simulink model "afe_abc_inv_psm"  (R2025b)
settings: Solver=ode1  StartTime=0.0  StopTime=simlength  FixedStep=tc  MaxStep=tc
values from neighbouring files (symbols this model uses):
  Adrso = eye(2) + Arso*ts_afe    [init_model.m]
  afe_pwm_phase_shift_mod1 = 0    [init_model.m]
  afe_pwm_phase_shift_mod2 = 0    [init_model.m]
  Aresd = eye(2) + Ares*ts_afe    [init_model.m]
  Bresd = Bres*ts_afe    [init_model.m]
  Cresd = Cres    [init_model.m]
  Crso = [1 0]    [init_model.m]
  CTRPIFF_CLIP_RELEASE = 0.001    [init_model.m]
  deepNEGeta = 0.5    [init_model.m]
  deepNEGxi = 0    [init_model.m]
  deepPOSxi = 0.5    [init_model.m]
  emf_fb_p = 0.2    [init_model.m]
  emf_fb_p_ccaller_1 = emf_fb_p    (= 0.2)    [init_model.m]
  emf_fb_p_ccaller_2 = emf_fb_p    (= 0.2)    [init_model.m]
  emf_p = emf_fb_p*4/10    (= 0.08)    [init_model.m]
  emf_p_ccaller_1 = emf_fb_p_ccaller_1*4/10    (= 0.08)    [init_model.m]
  emf_p_ccaller_2 = emf_fb_p_ccaller_2*4/10    (= 0.08)    [init_model.m]
  g0_161Hz = fcut_161Hz_flt * ts_afe * 2*pi    (= 0.126449104307)    [init_model.m]
  g0_1Hz = fcut_1Hz_flt * ts_afe * 2*pi    (= 0.000785398163397)    [init_model.m]
  g0_500Hz = fcut_500Hz_flt * ts_afe * 2*pi    (= 0.392699081699)    [init_model.m]
  g1_161Hz = 1 - g0_161Hz    (= 0.873550895693)    [init_model.m]
  g1_1Hz = 1 - g0_1Hz    (= 0.999214601837)    [init_model.m]
  g1_500Hz = 1 - g0_500Hz    (= 0.607300918301)    [init_model.m]
  i_grid_neg_eta_lim = 0.5    [init_model.m]
  i_grid_neg_eta_red_lim = 0.1    [init_model.m]
  i_grid_neg_xi_lim = 0.5    [init_model.m]
  i_grid_neg_xi_red_lim = 0.1    [init_model.m]
  i_grid_pos_eta_lim = 1    [init_model.m]
  i_grid_pos_eta_red_lim = 0.1    [init_model.m]
  id_lim = 0.35    [init_model.m]
  ieta_neg_ref_lim = 0.5    [init_model.m]
  ieta_pos_ref_lim = 1.0    (= 1)    [init_model.m]
  Igrid_phase_normalization_factor = 250e3/Vphase2/3/0.9*sqrt(2)    [init_model.m]
  inv_pwm_phase_shift_mod1 = 0    [init_model.m]
  iq_lim = 1.4    [init_model.m]
  ixi_pos_ref_lim = 1.6    [init_model.m]
  k_frt_ref = 2    [init_model.m]
  kg = Kobs(1)    [init_model.m]
  ki_afe = 45    [init_model.m]
  ki_align = 0.1    [init_model.m]
  ki_i = 18    [init_model.m]
  ki_rc_neg_grid = ki_rc_grid    (= 35)    [init_model.m]
  ki_rc_pos_grid = ki_rc_grid    (= 35)    [init_model.m]
  ki_vs = 35    [init_model.m]
  ki_w = 18    [init_model.m]
  kp_afe = 0.6    [init_model.m]
  kp_align = 0.6    [init_model.m]
  kp_i = 0.25    [init_model.m]
  kp_rc_neg_grid = kp_rc_grid    (= 0.35)    [init_model.m]
  kp_rc_pos_grid = kp_rc_grid    (= 0.35)    [init_model.m]
  kp_vs = 0.85    [init_model.m]
  kp_w = 2.5    [init_model.m]
  kw = Kobs(2)    [init_model.m]
  l1 = Kd(2)    [init_model.m]
  l2 = Kd(1)    [init_model.m]
  Ldrso = acker(Adrso',Crso',polesdrso)'    [init_model.m]
  lim_down_align = -0.2    [init_model.m]
  lim_up_align = 0.2    [init_model.m]
  mavarage_filter_frequency_base_order = 2    [init_model.m]
  motorc_m_scale = 2/3*Vdc_bez/ubez    [init_model.m]
  n1 = rms_perios/f_grid/ts_afe    [init_model.m]
  n10 = rms_perios/f_grid/ts_afe    [init_model.m]
  number_of_modules = 2    [init_model.m]
  omega_m_sim = omega_m_bez    [init_model.m]
  pll_i1 = 80    [init_model.m]
  pll_i1_ddsrt = pll_i1/2    (= 40)    [init_model.m]
  pll_p = 1    [init_model.m]
  pll_p_ddsrt = pll_p/2    (= 0.5)    [init_model.m]
  pll_p_frt = 0.2    [init_model.m]
  settle_time = 0.15    [init_model.m]
  simlength = 2    [init_model.m]
  start_time_LVRT = 2.0    (= 2)    [init_model.m]
  tc = ts_afe/200    (= 6.25e-07)    [init_model.m]
  time_aux_power_supply_fault = 1e3    (= 1000)    [init_model.m]
  time_gain_afe_module_1 = 1.0    (= 1)    [init_model.m]
  time_gain_afe_module_2 = 1.0    (= 1)    [init_model.m]
  time_gain_inv_module_1 = 1.0    (= 1)    [init_model.m]
  time_gain_inv_module_2 = 1.0    (= 1)    [init_model.m]
  time_phase_fault = 1e3    (= 1000)    [init_model.m]
  time_start_motor_control = 0.035    [init_model.m]
  transmission_delay = 125e-6*2    (= 0.00025)    [init_model.m]
  ts_afe = 1/fPWM_AFE/2    (= 0.000125)    [init_model.m]
  ts_inv = 1/fPWM_INV/2    (= 0.000125)    [init_model.m]
  Vdc_norm_ref = Vdc_ref/Vdc_nom    [init_model.m]
  Vdc_ref = 1070    [init_model.m]
  Vgrid_phase_normalization_factor = Vphase2*sqrt(2)    [init_model.m]
  w_grid = 2*pi*f_grid    [init_model.m]
undefined symbols (not defined in the file or in its folder): Amplitude_U, Amplitude_V, Amplitude_W, end_time_LVRT, ibez, La, Lb, Ld_norm, Lq_norm, Ls_norm, magnitude, omega_bez, omega_grid_emulator_nom, omega_grid_nom, omega_m_bez, Phase_shift, psi_bez, psi_m, psi_m_norm, rpm_base, rpm_bez, Rs, Rs_norm, t_ramp, tau_bez, torque_base, ubez, ugrid_factor, V_phase_normalization_factor, Vdc_bez, Vemu_ref_norm, vn_eta_pu, vn_xi_pu, vp_xi_pu
libraries: fl_lib x215, nesl_utility x107, simulink x22, cstblocks x20, threephase_inductor_lib x4, three_phase_pwm_modulator x4, single_phase_transformer_lib x3, power_meter_iec x1, flexshaft_lib x1, psm x1
(part 2 of 18)

== system afe_abc_inv_psm/afe_abc_inv_psm_mod1/brake ==
  Constant1 : Constant  Value=Vdc_ref
  Current Sensor3 : fl_lib/Electrical/Electrical Sensors/Current Sensor
  Integrator : Integrator
  MATLAB Function : MATLAB Function  TreatAsAtomicUnit=on  SystemSampleTime=ts_afe
  PS-Simulink Converter : nesl_utility/PS-Simulink Converter  PhysicalDomain=network_engine_domain  SubClassName=ps_output  LeftPortType=input  RightPortType=output  PseudoPeriodic=off  Frequencies=[]  VectorFormat=1-D array  Unit=V  AffineConversion=off
  Product : Product
  Product6 : Product
  Rbrake mod1 : Scope  NumInputPorts=2
      settings: SampleTime=tc  ActiveDisplayYMinimum=1.4840277431149421E-9  ActiveDisplayYMaximum=1.4991129263129132E-9  DataLoggingVariableName=ScopeData2
  Resistor : fl_lib/Electrical/Electrical Elements/Resistor  R=4 Ohm  i_specify=off  i_priority=None  i=0 A  i_nominal_specify=off  i_nominal_value=1  i_nominal_unit=A  v_specify=off  v_priority=None  v=0 V  v_nominal_specify=off  v_nominal_value=1  v_nominal_unit=V
  Simulink-PS Converter4 : nesl_utility/Simulink-PS Converter  PhysicalDomain=network_engine_domain  SubClassName=ps_input  LeftPortType=input  RightPortType=output  PseudoPeriodic=off  Frequencies=[]  NoiseDistribution=none  NoiseParameters=[]  Unit=1  AffineConversion=on  FilteringAndDerivatives=provide  SimscapeFilterOrder=1  InputFilterTimeConstant=0.001  UdotUserProvided=0
  Step : Step  Time=time_aux_power_supply_fault  Before=1  After=0  SampleTime=0
  To Workspace1 : ToWorkspace  VariableName=energy_Rbrake_sim_mod1  SampleTime=ts_afe
      settings: MaxDataPoints=Ns_afe
  To Workspace10 : ToWorkspace  VariableName=power_Rbrake_sim_mod1  SampleTime=ts_afe
      settings: MaxDataPoints=Ns_afe
  Unit Delay : UnitDelay  SampleTime=ts_afe  HasFrameUpgradeWarning=on
  Voltage Sensor : fl_lib/Electrical/Electrical Sensors/Voltage Sensor
  Voltage Sensor1 : fl_lib/Electrical/Electrical Sensors/Voltage Sensor
  ibrakeR : nesl_utility/PS-Simulink Converter  PhysicalDomain=network_engine_domain  SubClassName=ps_output  LeftPortType=input  RightPortType=output  PseudoPeriodic=off  Frequencies=[]  VectorFormat=1-D array  Unit=A  AffineConversion=off
  switch_5 : Subsystem
      settings: PortSchema="{\"entries\":[{\"content\":{\"sides\":[{\"content\":{\"connectorIds\":[\"LConn1\"]},\"type\":\"ConnectorPlacement.EquallySpacedRectSide\",\"uuid\":\"9277da8d-d460-43e6-8478-dd662f15d226\"},{\"content\":{\"connectorIds\":[],\"side\":\"RIGHT\"},\"type\":\"ConnectorPlacement.EquallySpacedRectSide\",\"uuid\":\"a7ece396-f1d9-4f4f-a05b-db1fc65d6e1d\"},{\"content\":{\"connectorIds\":[\"LConn2\"],\"side\":\"TOP\"},\"type\":\"ConnectorPlacement.EquallySpacedRectSide\",\"uuid\":\"fdd70777-e9cf-4317-afb6-cae87f75d5b0\"},{\"content\":{\"connectorIds\":[\"RConn1\"],\"side\":\"BOTTOM\"},\"type\":\"ConnectorPlacement.EquallySpacedRectSide\",\"uuid\":\"2353ed68-b1a1-4775-9ca9-31e268d5443b\"}]},\"type\":\"ConnectorPlacement.EquallySpacedConnector\",\"uuid\":\"d5479f4c-4e65-4791-adcb-73df11f88590\"}],\"packageUris\":[\"http://schema.mathworks.com/mf0/Connector/R2020b\"],\"version\":\"1.0\"}"
  switch_6 : Subsystem
      settings: PortSchema="{\"entries\":[{\"content\":{\"sides\":[{\"content\":{},\"type\":\"ConnectorPlacement.EquallySpacedRectSide\",\"uuid\":\"9277da8d-d460-43e6-8478-dd662f15d226\"},{\"content\":{\"side\":\"RIGHT\"},\"type\":\"ConnectorPlacement.EquallySpacedRectSide\",\"uuid\":\"a7ece396-f1d9-4f4f-a05b-db1fc65d6e1d\"},{\"content\":{\"connectorIds\":[\"LConn1\"],\"side\":\"TOP\"},\"type\":\"ConnectorPlacement.EquallySpacedRectSide\",\"uuid\":\"fdd70777-e9cf-4317-afb6-cae87f75d5b0\"},{\"content\":{\"connectorIds\":[\"RConn1\"],\"side\":\"BOTTOM\"},\"type\":\"ConnectorPlacement.EquallySpacedRectSide\",\"uuid\":\"2353ed68-b1a1-4775-9ca9-31e268d5443b\"}]},\"type\":\"ConnectorPlacement.EquallySpacedConnector\",\"uuid\":\"d5479f4c-4e65-4791-adcb-73df11f88590\"}],\"packageUris\":[\"http://schema.mathworks.com/mf0/Connector/R2020b\"],\"version\":\"1.0\"}"
  ubrakeR : nesl_utility/PS-Simulink Converter  PhysicalDomain=network_engine_domain  SubClassName=ps_output  LeftPortType=input  RightPortType=output  PseudoPeriodic=off  Frequencies=[]  VectorFormat=1-D array  Unit=V  AffineConversion=off
  dc(+) : PMIOPort  Side=Left
  dc(-) : PMIOPort  Port=2  Side=Left
  tag scope: energy_Rbrake_mod1=global, power_Rbrake_mod1=global
  wires:
  Constant1/1 -> MATLAB Function/2(udc_ref)
  PS-Simulink Converter/1 -> MATLAB Function/1(u)
  MATLAB Function/1(y) -> Unit Delay/1
  ibrakeR/1 -> Product/1  "ibrakeR"
  ubrakeR/1 -> Product/2  "ubrakeR"
  Product/1 -> [power_Rbrake_mod1], Integrator/1
  Integrator/1 -> [energy_Rbrake_mod1]
  [power_Rbrake_mod1] -> To Workspace10/1, Rbrake mod1/1  "power_Rbrake"
  [energy_Rbrake_mod1] -> To Workspace1/1, Rbrake mod1/2  "energy_Rbrake"
  Step/1 -> Product6/1
  Unit Delay/1 -> Product6/2
  Product6/1 -> Simulink-PS Converter4/1
  connections:
  dc(-)/RConn1 -- switch_5/RConn1 -- Voltage Sensor/RConn2
  Voltage Sensor1/LConn1 -- Resistor/LConn1 -- Current Sensor3/RConn2
  PS-Simulink Converter/LConn1 -- Voltage Sensor/RConn1
  switch_5/LConn1 -- Simulink-PS Converter4/RConn1
  switch_6/RConn1 -- Voltage Sensor1/RConn2 -- Resistor/RConn1 -- switch_5/LConn2
  Voltage Sensor/LConn1 -- Current Sensor3/LConn1 -- switch_6/LConn1 -- dc(+)/RConn1
  Current Sensor3/RConn1 -- ibrakeR/LConn1
  Voltage Sensor1/RConn1 -- ubrakeR/LConn1

== system afe_abc_inv_psm/afe_abc_inv_psm_mod1/inverter ==
  duvw : Inport
  Current Sensor : fl_lib/Electrical/Electrical Sensors/Current Sensor
  PS-Simulink Converter1 : nesl_utility/PS-Simulink Converter  PhysicalDomain=network_engine_domain  SubClassName=ps_output  LeftPortType=input  RightPortType=output  PseudoPeriodic=off  Frequencies=[]  VectorFormat=1-D array  Unit=A  AffineConversion=on
  PS-Simulink Converter4 : nesl_utility/PS-Simulink Converter  PhysicalDomain=network_engine_domain  SubClassName=ps_output  LeftPortType=input  RightPortType=output  PseudoPeriodic=off  Frequencies=[]  VectorFormat=1-D array  Unit=V  AffineConversion=on
  To Workspace : ToWorkspace  VariableName=idc_sim_mod1  SampleTime=tc
      settings: MaxDataPoints=Nc
  To Workspace1 : ToWorkspace  VariableName=udc_sim_mod1  SampleTime=tc
      settings: MaxDataPoints=Nc
  Transfer Fcn : TransferFcn  Denominator=[1e-2 1]
  Voltage Sensor : fl_lib/Electrical/Electrical Sensors/Voltage Sensor
  idc/udc : Scope  NumInputPorts=2
      settings: SampleTime=tc  ActiveDisplayYMinimum=-232.79227304961765  ActiveDisplayYMaximum=27.545875945686063
  inverter : Subsystem
  Udc(+) : PMIOPort  Side=Right
  Udc(-) : PMIOPort  Port=2  Side=Right
  us_u : PMIOPort  Port=3  Side=Left
  us_v : PMIOPort  Port=4  Side=Left
  us_w : PMIOPort  Port=5  Side=Left
  wires:
  PS-Simulink Converter4/1 -> To Workspace1/1, idc/udc/2  "udc"
  PS-Simulink Converter1/1 -> Transfer Fcn/1  "idc"
  Transfer Fcn/1 -> To Workspace/1, idc/udc/1  "idc_flt"
  duvw/1 -> inverter/1(duties_uvw)
  connections:
  PS-Simulink Converter4/LConn1 -- Voltage Sensor/RConn1
  us_u/RConn1 -- inverter/LConn1
  us_v/RConn1 -- inverter/LConn2
  us_w/RConn1 -- inverter/LConn3
  Voltage Sensor/RConn2 -- inverter/RConn2 -- Udc(-)/RConn1
  Current Sensor/LConn1 -- Udc(+)/RConn1
  Voltage Sensor/LConn1 -- inverter/RConn1 -- Current Sensor/RConn2
  PS-Simulink Converter1/LConn1 -- Current Sensor/RConn1

== system afe_abc_inv_psm/afe_abc_inv_psm_mod2/AFE_control ==
  afe_control : Subsystem
  dabc_out : Outport
  tag scope: local_time_corr_afe2=global
  wires:
  [ig_abc_pu_mod2] -> afe_control/3(ig_abc_pu)
  afe_control/1(duvw) -> dabc_out/1
  [vdc_pu_afe_mod2] -> afe_control/2(udc_pu)
  [is_abc_pu_mod2] -> afe_control/4(is_abc_pu)
  [ug_abc_pu_mod2] -> afe_control/1(ug_abc_pu)
  [TRGO_afe_module_2] -> afe_control/Trigger
  [time_afe_module_2] -> afe_control/5(local_time)
  [time_master] -> afe_control/6(master_time)
  afe_control/2(AFE2_local_time_corr) -> [local_time_corr_afe2]

== system afe_abc_inv_psm/afe_abc_inv_psm_mod2/INV_control ==
  inverter_control : Subsystem
  transmission_delay : UnitDelay  SampleTime=transmission_delay  HasFrameUpgradeWarning=on
  duvw_out : Outport
  tag scope: local_time_corr_inv2=global
  wires:
  inverter_control/1(duvw) -> duvw_out/1
  [vdc_pu_inv_mod2] -> inverter_control/2(udc_pu)
  [TRGO_inv_module_2] -> inverter_control/Trigger
  [is_uvw_pu_mod2] -> inverter_control/1(is_uvw)
  [time_inv_module_2] -> inverter_control/3(local_time)
  [time_master] -> inverter_control/4(master_time)
  inverter_control/2(INV2_local_time_corr) -> [local_time_corr_inv2]
  [master_torque_ref] -> transmission_delay/1
  transmission_delay/1 -> inverter_control/5(master_torque_ref)
  [theta_elec_psm] -> inverter_control/6(theta_elec_psm)

== system afe_abc_inv_psm/afe_abc_inv_psm_mod2/LCL_filter ==
  CFu1 : fl_lib/Electrical/Electrical Elements/Capacitor  c=CFu F  r=RCFu Ohm  g=0 1/Ohm  i_specify=off  i_priority=None  i=0 A  i_nominal_specify=off  i_nominal_value=1  i_nominal_unit=A  v_specify=off  v_priority=None  v=0 V  v_nominal_specify=off  v_nominal_value=1  v_nominal_unit=V  vc_specify=off  vc_priority=High  vc=0 V  vc_nominal_specify=off  vc_nominal_value=1  vc_nominal_unit=V
  CFu2 : fl_lib/Electrical/Electrical Elements/Capacitor  c=CFu F  r=RCFu Ohm  g=0 1/Ohm  i_specify=off  i_priority=None  i=0 A  i_nominal_specify=off  i_nominal_value=1  i_nominal_unit=A  v_specify=off  v_priority=None  v=0 V  v_nominal_specify=off  v_nominal_value=1  v_nominal_unit=V  vc_specify=off  vc_priority=High  vc=0 V  vc_nominal_specify=off  vc_nominal_value=1  vc_nominal_unit=V
  CFu3 : fl_lib/Electrical/Electrical Elements/Capacitor  c=CFu F  r=RCFu Ohm  g=0 1/Ohm  i_specify=off  i_priority=None  i=0 A  i_nominal_specify=off  i_nominal_value=1  i_nominal_unit=A  v_specify=off  v_priority=None  v=0 V  v_nominal_specify=off  v_nominal_value=1  v_nominal_unit=V  vc_specify=off  vc_priority=High  vc=0 V  vc_nominal_specify=off  vc_nominal_value=1  vc_nominal_unit=V
  Inductor : fl_lib/Electrical/Electrical Elements/Inductor  l=1e-6 H  r=0 Ohm  g=1e-9 1/Ohm  i_specify=on  i_priority=High  i=0 A  i_nominal_specify=off  i_nominal_value=1  i_nominal_unit=A  v_specify=off  v_priority=None  v=0 V  v_nominal_specify=off  v_nominal_value=1  v_nominal_unit=V  i_L_specify=off  i_L_priority=High  i_L=0 A  i_L_nominal_specify=off  i_L_nominal_value=1  i_L_nominal_unit=A
  Inductor1 : fl_lib/Electrical/Electrical Elements/Inductor  l=1e-6 H  r=0 Ohm  g=1e-9 1/Ohm  i_specify=on  i_priority=High  i=0 A  i_nominal_specify=off  i_nominal_value=1  i_nominal_unit=A  v_specify=off  v_priority=None  v=0 V  v_nominal_specify=off  v_nominal_value=1  v_nominal_unit=V  i_L_specify=off  i_L_priority=High  i_L=0 A  i_L_nominal_specify=off  i_L_nominal_value=1  i_L_nominal_unit=A
  Inductor2 : fl_lib/Electrical/Electrical Elements/Inductor  l=1e-6 H  r=0 Ohm  g=1e-9 1/Ohm  i_specify=on  i_priority=High  i=0 A  i_nominal_specify=off  i_nominal_value=1  i_nominal_unit=A  v_specify=off  v_priority=None  v=0 V  v_nominal_specify=off  v_nominal_value=1  v_nominal_unit=V  i_L_specify=off  i_L_priority=High  i_L=0 A  i_L_nominal_specify=off  i_L_nominal_value=1  i_L_nominal_unit=A
  threephase inductor : threephase_inductor_lib/threephase inductor  Lp=LFu1_AFE H  L0=LFu1_AFE_0 H  Rp=2.4e-3 Ohm  R0=0.8e-3 Ohm  Lls=5e-6 H  uu_1_specify=off  uu_1_priority=None  uu_1=0 V  uu_1_nominal_specify=off  uu_1_nominal_unit=V  uu_1_nominal_value=1  uv_1_specify=off  uv_1_priority=None  uv_1=0 V  uv_1_nominal_specify=off  uv_1_nominal_unit=V  uv_1_nominal_value=1  uw_1_specify=off  uw_1_priority=None  uw_1=0 V  uw_1_nominal_specify=off  uw_1_nominal_unit=V  uw_1_nominal_value=1  uu_2_specify=off  uu_2_priority=None  uu_2=0 V  uu_2_nominal_specify=off  uu_2_nominal_unit=V  uu_2_nominal_value=1  uv_2_specify=off  uv_2_priority=None  uv_2=0 V  uv_2_nominal_specify=off  uv_2_nominal_unit=V  uv_2_nominal_value=1  uw_2_specify=off  uw_2_priority=None  uw_2=0 V  uw_2_nominal_specify=off  uw_2_nominal_unit=V  uw_2_nominal_value=1  iu_specify=off  iu_priority=High  iu=0 A  iu_nominal_specify=off  iu_nominal_unit=A  iu_nominal_value=1  iv_specify=off  iv_priority=High  iv=0 A  iv_nominal_specify=off  iv_nominal_unit=A  iv_nominal_value=1  iw_specify=off  iw_priority=High  iw=0 A  iw_nominal_specify=off  iw_nominal_unit=A  iw_nominal_value=1
      settings: InternalSimscapePortConfiguration="{\"Bottom\":[],\"Left\":[{\"id\":\"up1\",\"label\":\"u1\",\"type\":\"foundation.electrical.electrical\"},{\"id\":\"vp1\",\"label\":\"v1\",\"type\":\"foundation.electrical.electrical\"},{\"id\":\"wp1\",\"label\":\"w1\",\"type\":\"foundation.electrical.electrical\"}],\"Right\":[{\"id\":\"up2\",\"label\":\"u2\",\"type\":\"foundation.electrical.electrical\"},{\"id\":\"vp2\",\"label\":\"v2\",\"type\":\"foundation.electrical.electrical\"},{\"id\":\"wp2\",\"label\":\"w2\",\"type\":\"foundation.electrical.electrical\"}],\"Top\":[]}"
  threephase_vi_measures_stack : Subsystem
  threephase_vi_measures_stack1 : Subsystem
  us_a : PMIOPort  Side=Left
  ug_a : PMIOPort  Port=2  Side=Right
  us_b : PMIOPort  Port=3  Side=Left
  ug_b : PMIOPort  Port=4  Side=Right
  us_c : PMIOPort  Port=5  Side=Left
  ug_c : PMIOPort  Port=6  Side=Right
  connections:
  ug_c/RConn1 -- threephase_vi_measures_stack1/RConn3
  ug_b/RConn1 -- threephase_vi_measures_stack1/RConn2
  ug_a/RConn1 -- threephase_vi_measures_stack1/RConn1
  Inductor2/LConn1 -- threephase inductor/RConn3
  Inductor1/LConn1 -- threephase inductor/RConn2
  threephase inductor/RConn1 -- Inductor/LConn1
  threephase_vi_measures_stack/RConn3 -- threephase inductor/LConn3
  threephase_vi_measures_stack/RConn2 -- threephase inductor/LConn2
  threephase_vi_measures_stack/RConn1 -- threephase inductor/LConn1
  threephase_vi_measures_stack/LConn3 -- us_c/RConn1
  threephase_vi_measures_stack/LConn2 -- us_b/RConn1
  threephase_vi_measures_stack/LConn1 -- us_a/RConn1
  CFu2/LConn1 -- threephase_vi_measures_stack1/LConn2 -- Inductor1/RConn1
  CFu3/LConn1 -- threephase_vi_measures_stack1/LConn3 -- Inductor2/RConn1
  CFu1/LConn1 -- threephase_vi_measures_stack1/LConn1 -- Inductor/RConn1
  CFu1/RConn1 -- CFu2/RConn1 -- CFu3/RConn1

== system afe_abc_inv_psm/afe_abc_inv_psm_mod2/L_filter ==
  Inductor : fl_lib/Electrical/Electrical Elements/Inductor  l=1e-6 H  r=0 Ohm  g=1e-9 1/Ohm  i_specify=off  i_priority=None  i=0 A  i_nominal_specify=off  i_nominal_value=1  i_nominal_unit=A  v_specify=off  v_priority=None  v=0 V  v_nominal_specify=off  v_nominal_value=1  v_nominal_unit=V  i_L_specify=off  i_L_priority=High  i_L=0 A  i_L_nominal_specify=off  i_L_nominal_value=1  i_L_nominal_unit=A
  Inductor1 : fl_lib/Electrical/Electrical Elements/Inductor  l=1e-6 H  r=0 Ohm  g=1e-9 1/Ohm  i_specify=off  i_priority=None  i=0 A  i_nominal_specify=off  i_nominal_value=1  i_nominal_unit=A  v_specify=off  v_priority=None  v=0 V  v_nominal_specify=off  v_nominal_value=1  v_nominal_unit=V  i_L_specify=off  i_L_priority=High  i_L=0 A  i_L_nominal_specify=off  i_L_nominal_value=1  i_L_nominal_unit=A
  Inductor2 : fl_lib/Electrical/Electrical Elements/Inductor  l=1e-6 H  r=0 Ohm  g=1e-9 1/Ohm  i_specify=off  i_priority=None  i=0 A  i_nominal_specify=off  i_nominal_value=1  i_nominal_unit=A  v_specify=off  v_priority=None  v=0 V  v_nominal_specify=off  v_nominal_value=1  v_nominal_unit=V  i_L_specify=off  i_L_priority=High  i_L=0 A  i_L_nominal_specify=off  i_L_nominal_value=1  i_L_nominal_unit=A
  threephase inductor : threephase_inductor_lib/threephase inductor  Lp=LFi H  L0=LFi_0 H  Rp=2.4e-3 Ohm  R0=0.8e-3 Ohm  Lls=5e-6 H  uu_1_specify=off  uu_1_priority=None  uu_1=0 V  uu_1_nominal_specify=off  uu_1_nominal_unit=V  uu_1_nominal_value=1  uv_1_specify=off  uv_1_priority=None  uv_1=0 V  uv_1_nominal_specify=off  uv_1_nominal_unit=V  uv_1_nominal_value=1  uw_1_specify=off  uw_1_priority=None  uw_1=0 V  uw_1_nominal_specify=off  uw_1_nominal_unit=V  uw_1_nominal_value=1  uu_2_specify=off  uu_2_priority=None  uu_2=0 V  uu_2_nominal_specify=off  uu_2_nominal_unit=V  uu_2_nominal_value=1  uv_2_specify=off  uv_2_priority=None  uv_2=0 V  uv_2_nominal_specify=off  uv_2_nominal_unit=V  uv_2_nominal_value=1  uw_2_specify=off  uw_2_priority=None  uw_2=0 V  uw_2_nominal_specify=off  uw_2_nominal_unit=V  uw_2_nominal_value=1  iu_specify=off  iu_priority=None  iu=0 A  iu_nominal_specify=off  iu_nominal_unit=A  iu_nominal_value=1  iv_specify=off  iv_priority=None  iv=0 A  iv_nominal_specify=off  iv_nominal_unit=A  iv_nominal_value=1  iw_specify=off  iw_priority=None  iw=0 A  iw_nominal_specify=off  iw_nominal_unit=A  iw_nominal_value=1
      settings: InternalSimscapePortConfiguration="{\"Bottom\":[],\"Left\":[{\"id\":\"up1\",\"label\":\"u1\",\"type\":\"foundation.electrical.electrical\"},{\"id\":\"vp1\",\"label\":\"v1\",\"type\":\"foundation.electrical.electrical\"},{\"id\":\"wp1\",\"label\":\"w1\",\"type\":\"foundation.electrical.electrical\"}],\"Right\":[{\"id\":\"up2\",\"label\":\"u2\",\"type\":\"foundation.electrical.electrical\"},{\"id\":\"vp2\",\"label\":\"v2\",\"type\":\"foundation.electrical.electrical\"},{\"id\":\"wp2\",\"label\":\"w2\",\"type\":\"foundation.electrical.electrical\"}],\"Top\":[]}"
  threephase_vi_measures_stack : Subsystem
  us_u : PMIOPort  Side=Left
  uu : PMIOPort  Port=2  Side=Right
  us_v : PMIOPort  Port=3  Side=Left
  uv : PMIOPort  Port=4  Side=Right
  us_w : PMIOPort  Port=5  Side=Left
  uw : PMIOPort  Port=6  Side=Right
  connections:
  Inductor2/RConn1 -- uw/RConn1
  Inductor1/RConn1 -- uv/RConn1
  Inductor/RConn1 -- uu/RConn1
  threephase inductor/RConn3 -- Inductor2/LConn1
  threephase inductor/RConn2 -- Inductor1/LConn1
  threephase inductor/RConn1 -- Inductor/LConn1
  threephase inductor/LConn3 -- threephase_vi_measures_stack/RConn3
  threephase inductor/LConn2 -- threephase_vi_measures_stack/RConn2
  threephase inductor/LConn1 -- threephase_vi_measures_stack/RConn1
  threephase_vi_measures_stack/LConn3 -- us_w/RConn1
  threephase_vi_measures_stack/LConn2 -- us_v/RConn1
  threephase_vi_measures_stack/LConn1 -- us_u/RConn1

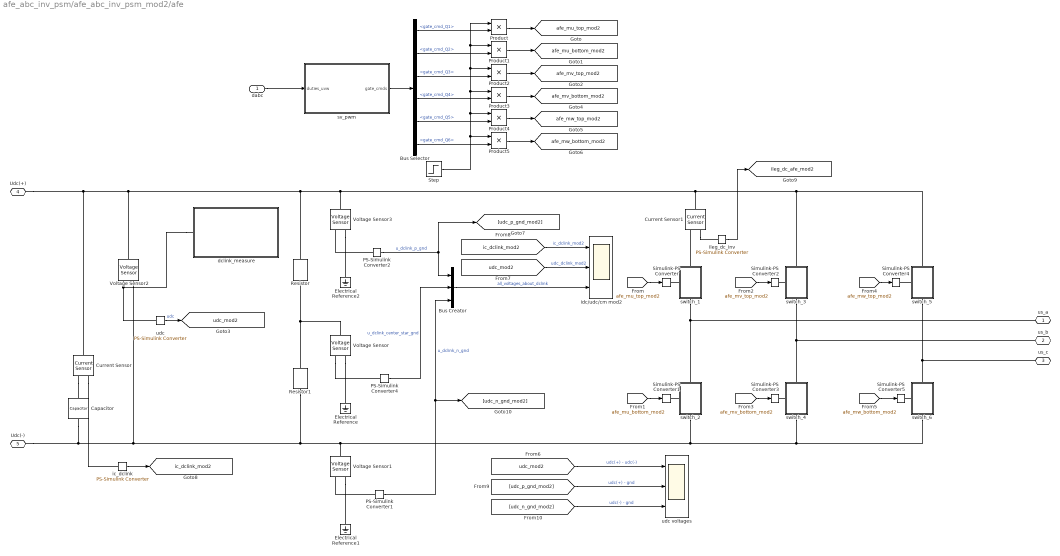
== system afe_abc_inv_psm/afe_abc_inv_psm_mod2/afe ==
  dabc : Inport
  Bus Creator : BusCreator  Inputs=3
  Bus Selector : BusSelector  OutputSignals=gate_cmd_Q1,gate_cmd_Q2,gate_cmd_Q3,gate_cmd_Q4,gate_cmd_Q5,gate_cmd_Q6
  Capacitor : fl_lib/Electrical/Electrical Elements/Capacitor  c=CFi F  r=0.2e-3 Ohm  g=0 1/Ohm  i_specify=off  i_priority=None  i=0 A  i_nominal_specify=off  i_nominal_value=1  i_nominal_unit=A  v_specify=on  v_priority=High  v=Vdc_bez V  v_nominal_specify=off  v_nominal_value=1  v_nominal_unit=V  vc_specify=on  vc_priority=High  vc=Vdc_bez V  vc_nominal_specify=off  vc_nominal_value=1  vc_nominal_unit=V
  Current Sensor : fl_lib/Electrical/Electrical Sensors/Current Sensor
  Current Sensor1 : fl_lib/Electrical/Electrical Sensors/Current Sensor
  Electrical Reference : fl_lib/Electrical/Electrical Elements/Electrical Reference
  Electrical Reference1 : fl_lib/Electrical/Electrical Elements/Electrical Reference
  Electrical Reference2 : fl_lib/Electrical/Electrical Elements/Electrical Reference
  PS-Simulink Converter1 : nesl_utility/PS-Simulink Converter  PhysicalDomain=network_engine_domain  SubClassName=ps_output  LeftPortType=input  RightPortType=output  PseudoPeriodic=off  Frequencies=[]  VectorFormat=1-D array  Unit=V  AffineConversion=on
  PS-Simulink Converter2 : nesl_utility/PS-Simulink Converter  PhysicalDomain=network_engine_domain  SubClassName=ps_output  LeftPortType=input  RightPortType=output  PseudoPeriodic=off  Frequencies=[]  VectorFormat=1-D array  Unit=V  AffineConversion=on
  PS-Simulink Converter4 : nesl_utility/PS-Simulink Converter  PhysicalDomain=network_engine_domain  SubClassName=ps_output  LeftPortType=input  RightPortType=output  PseudoPeriodic=off  Frequencies=[]  VectorFormat=1-D array  Unit=V  AffineConversion=on
  Product{,1..5} (6 alike) : Product
  Resistor : fl_lib/Electrical/Electrical Elements/Resistor  R=1e6 Ohm  i_specify=off  i_priority=None  i=0 A  i_nominal_specify=off  i_nominal_value=1  i_nominal_unit=A  v_specify=off  v_priority=None  v=0 V  v_nominal_specify=off  v_nominal_value=1  v_nominal_unit=V
  Resistor1 : fl_lib/Electrical/Electrical Elements/Resistor  R=1e6 Ohm  i_specify=off  i_priority=None  i=0 A  i_nominal_specify=off  i_nominal_value=1  i_nominal_unit=A  v_specify=off  v_priority=None  v=0 V  v_nominal_specify=off  v_nominal_value=1  v_nominal_unit=V
  Simulink-PS Converter{,1..5} (6 alike) : nesl_utility/Simulink-PS Converter  PhysicalDomain=network_engine_domain  SubClassName=ps_input  LeftPortType=input  RightPortType=output  PseudoPeriodic=off  Frequencies=[]  NoiseDistribution=none  NoiseParameters=[]  Unit=1  AffineConversion=off  FilteringAndDerivatives=provide  SimscapeFilterOrder=1  InputFilterTimeConstant=0.001  UdotUserProvided=0
  Step : Step  Time=time_aux_power_supply_fault  Before=1  After=0  SampleTime=0
  Voltage Sensor{,1..3} (4 alike) : fl_lib/Electrical/Electrical Sensors/Voltage Sensor
  dclink_measure : Subsystem
  ic_dclink : nesl_utility/PS-Simulink Converter  PhysicalDomain=network_engine_domain  SubClassName=ps_output  LeftPortType=input  RightPortType=output  PseudoPeriodic=off  Frequencies=[]  VectorFormat=1-D array  Unit=A  AffineConversion=on
  idc/udc/cm mod2 : Scope  NumInputPorts=3
      settings: SampleTime=tc  ActiveDisplayYMinimum=-429.54161859669227  ActiveDisplayYMaximum=384.63505854745779
  ileg_dc_inv : nesl_utility/PS-Simulink Converter  PhysicalDomain=network_engine_domain  SubClassName=ps_output  LeftPortType=input  RightPortType=output  PseudoPeriodic=off  Frequencies=[]  VectorFormat=1-D array  Unit=A  AffineConversion=on
  sv_pwm : Subsystem
  switch_1 : Subsystem
      settings: PortSchema="{\"entries\":[{\"content\":{\"sides\":[{\"content\":{\"connectorIds\":[\"LConn1\"]},\"type\":\"ConnectorPlacement.EquallySpacedRectSide\",\"uuid\":\"9277da8d-d460-43e6-8478-dd662f15d226\"},{\"content\":{\"connectorIds\":[],\"side\":\"RIGHT\"},\"type\":\"ConnectorPlacement.EquallySpacedRectSide\",\"uuid\":\"a7ece396-f1d9-4f4f-a05b-db1fc65d6e1d\"},{\"content\":{\"connectorIds\":[\"LConn2\"],\"side\":\"TOP\"},\"type\":\"ConnectorPlacement.EquallySpacedRectSide\",\"uuid\":\"fdd70777-e9cf-4317-afb6-cae87f75d5b0\"},{\"content\":{\"connectorIds\":[\"RConn1\"],\"side\":\"BOTTOM\"},\"type\":\"ConnectorPlacement.EquallySpacedRectSide\",\"uuid\":\"2353ed68-b1a1-4775-9ca9-31e268d5443b\"}]},\"type\":\"ConnectorPlacement.EquallySpacedConnector\",\"uuid\":\"d5479f4c-4e65-4791-adcb-73df11f88590\"}],\"packageUris\":[\"http://schema.mathworks.com/mf0/Connector/R2020b\"],\"version\":\"1.0\"}"
  switch_2 : Subsystem
      settings: PortSchema="{\"entries\":[{\"content\":{\"sides\":[{\"content\":{\"connectorIds\":[\"LConn1\"]},\"type\":\"ConnectorPlacement.EquallySpacedRectSide\",\"uuid\":\"9277da8d-d460-43e6-8478-dd662f15d226\"},{\"content\":{\"connectorIds\":[],\"side\":\"RIGHT\"},\"type\":\"ConnectorPlacement.EquallySpacedRectSide\",\"uuid\":\"a7ece396-f1d9-4f4f-a05b-db1fc65d6e1d\"},{\"content\":{\"connectorIds\":[\"LConn2\"],\"side\":\"TOP\"},\"type\":\"ConnectorPlacement.EquallySpacedRectSide\",\"uuid\":\"fdd70777-e9cf-4317-afb6-cae87f75d5b0\"},{\"content\":{\"connectorIds\":[\"RConn1\"],\"side\":\"BOTTOM\"},\"type\":\"ConnectorPlacement.EquallySpacedRectSide\",\"uuid\":\"2353ed68-b1a1-4775-9ca9-31e268d5443b\"}]},\"type\":\"ConnectorPlacement.EquallySpacedConnector\",\"uuid\":\"d5479f4c-4e65-4791-adcb-73df11f88590\"}],\"packageUris\":[\"http://schema.mathworks.com/mf0/Connector/R2020b\"],\"version\":\"1.0\"}"
  switch_3 : Subsystem
      settings: PortSchema="{\"entries\":[{\"content\":{\"sides\":[{\"content\":{\"connectorIds\":[\"LConn1\"]},\"type\":\"ConnectorPlacement.EquallySpacedRectSide\",\"uuid\":\"9277da8d-d460-43e6-8478-dd662f15d226\"},{\"content\":{\"connectorIds\":[],\"side\":\"RIGHT\"},\"type\":\"ConnectorPlacement.EquallySpacedRectSide\",\"uuid\":\"a7ece396-f1d9-4f4f-a05b-db1fc65d6e1d\"},{\"content\":{\"connectorIds\":[\"LConn2\"],\"side\":\"TOP\"},\"type\":\"ConnectorPlacement.EquallySpacedRectSide\",\"uuid\":\"fdd70777-e9cf-4317-afb6-cae87f75d5b0\"},{\"content\":{\"connectorIds\":[\"RConn1\"],\"side\":\"BOTTOM\"},\"type\":\"ConnectorPlacement.EquallySpacedRectSide\",\"uuid\":\"2353ed68-b1a1-4775-9ca9-31e268d5443b\"}]},\"type\":\"ConnectorPlacement.EquallySpacedConnector\",\"uuid\":\"d5479f4c-4e65-4791-adcb-73df11f88590\"}],\"packageUris\":[\"http://schema.mathworks.com/mf0/Connector/R2020b\"],\"version\":\"1.0\"}"
  switch_4 : Subsystem
      settings: PortSchema="{\"entries\":[{\"content\":{\"sides\":[{\"content\":{\"connectorIds\":[\"LConn1\"]},\"type\":\"ConnectorPlacement.EquallySpacedRectSide\",\"uuid\":\"9277da8d-d460-43e6-8478-dd662f15d226\"},{\"content\":{\"connectorIds\":[],\"side\":\"RIGHT\"},\"type\":\"ConnectorPlacement.EquallySpacedRectSide\",\"uuid\":\"a7ece396-f1d9-4f4f-a05b-db1fc65d6e1d\"},{\"content\":{\"connectorIds\":[\"LConn2\"],\"side\":\"TOP\"},\"type\":\"ConnectorPlacement.EquallySpacedRectSide\",\"uuid\":\"fdd70777-e9cf-4317-afb6-cae87f75d5b0\"},{\"content\":{\"connectorIds\":[\"RConn1\"],\"side\":\"BOTTOM\"},\"type\":\"ConnectorPlacement.EquallySpacedRectSide\",\"uuid\":\"2353ed68-b1a1-4775-9ca9-31e268d5443b\"}]},\"type\":\"ConnectorPlacement.EquallySpacedConnector\",\"uuid\":\"d5479f4c-4e65-4791-adcb-73df11f88590\"}],\"packageUris\":[\"http://schema.mathworks.com/mf0/Connector/R2020b\"],\"version\":\"1.0\"}"
  switch_5 : Subsystem
      settings: PortSchema="{\"entries\":[{\"content\":{\"sides\":[{\"content\":{\"connectorIds\":[\"LConn1\"]},\"type\":\"ConnectorPlacement.EquallySpacedRectSide\",\"uuid\":\"9277da8d-d460-43e6-8478-dd662f15d226\"},{\"content\":{\"connectorIds\":[],\"side\":\"RIGHT\"},\"type\":\"ConnectorPlacement.EquallySpacedRectSide\",\"uuid\":\"a7ece396-f1d9-4f4f-a05b-db1fc65d6e1d\"},{\"content\":{\"connectorIds\":[\"LConn2\"],\"side\":\"TOP\"},\"type\":\"ConnectorPlacement.EquallySpacedRectSide\",\"uuid\":\"fdd70777-e9cf-4317-afb6-cae87f75d5b0\"},{\"content\":{\"connectorIds\":[\"RConn1\"],\"side\":\"BOTTOM\"},\"type\":\"ConnectorPlacement.EquallySpacedRectSide\",\"uuid\":\"2353ed68-b1a1-4775-9ca9-31e268d5443b\"}]},\"type\":\"ConnectorPlacement.EquallySpacedConnector\",\"uuid\":\"d5479f4c-4e65-4791-adcb-73df11f88590\"}],\"packageUris\":[\"http://schema.mathworks.com/mf0/Connector/R2020b\"],\"version\":\"1.0\"}"
  switch_6 : Subsystem
      settings: PortSchema="{\"entries\":[{\"content\":{\"sides\":[{\"content\":{\"connectorIds\":[\"LConn1\"]},\"type\":\"ConnectorPlacement.EquallySpacedRectSide\",\"uuid\":\"9277da8d-d460-43e6-8478-dd662f15d226\"},{\"content\":{\"connectorIds\":[],\"side\":\"RIGHT\"},\"type\":\"ConnectorPlacement.EquallySpacedRectSide\",\"uuid\":\"a7ece396-f1d9-4f4f-a05b-db1fc65d6e1d\"},{\"content\":{\"connectorIds\":[\"LConn2\"],\"side\":\"TOP\"},\"type\":\"ConnectorPlacement.EquallySpacedRectSide\",\"uuid\":\"fdd70777-e9cf-4317-afb6-cae87f75d5b0\"},{\"content\":{\"connectorIds\":[\"RConn1\"],\"side\":\"BOTTOM\"},\"type\":\"ConnectorPlacement.EquallySpacedRectSide\",\"uuid\":\"2353ed68-b1a1-4775-9ca9-31e268d5443b\"}]},\"type\":\"ConnectorPlacement.EquallySpacedConnector\",\"uuid\":\"d5479f4c-4e65-4791-adcb-73df11f88590\"}],\"packageUris\":[\"http://schema.mathworks.com/mf0/Connector/R2020b\"],\"version\":\"1.0\"}"
  udc : nesl_utility/PS-Simulink Converter  PhysicalDomain=network_engine_domain  SubClassName=ps_output  LeftPortType=input  RightPortType=output  PseudoPeriodic=off  Frequencies=[]  VectorFormat=1-D array  Unit=V  AffineConversion=on
  udc voltages : Scope  NumInputPorts=3
      settings: SampleTime=tc  ActiveDisplayYMinimum=965.52412499575871  ActiveDisplayYMaximum=1296.0343915128553
  us_a : PMIOPort  Side=Left
  us_b : PMIOPort  Port=2  Side=Left
  us_c : PMIOPort  Port=3  Side=Left
  Udc(+) : PMIOPort  Port=4  Side=Right
  Udc(-) : PMIOPort  Port=5  Side=Right
  tag scope: afe_mu_bottom_mod2=global, afe_mu_top_mod2=global, afe_mv_bottom_mod2=global, afe_mv_top_mod2=global, afe_mw_bottom_mod2=global, afe_mw_top_mod2=global, ic_dclink_mod2=global, ileg_dc_afe_mod2=global, udc_mod2=global
  wires:
  [udc_mod2] -> udc voltages/1  "udc(+) - udc(-)"
  [udc_n_gnd_mod2] -> udc voltages/3  "udc(-) - gnd"
  [udc_p_gnd_mod2] -> udc voltages/2  "udc(+) - gnd"
  PS-Simulink Converter1/1 -> [udc_n_gnd_mod2], Bus Creator/3  "u_dclink_n_gnd"
  PS-Simulink Converter4/1 -> Bus Creator/2  "u_dclink_center_star_gnd"
  PS-Simulink Converter2/1 -> Bus Creator/1, [udc_p_gnd_mod2]  "u_dclink_p_gnd"
  Bus Creator/1 -> idc/udc/cm mod2/3  "all_voltages_about_dclink"
  [udc_mod2] -> idc/udc/cm mod2/2  "udc_dclink_mod2"
  [ic_dclink_mod2] -> idc/udc/cm mod2/1  "ic_dclink_mod2"
  Product5/1 -> [afe_mw_bottom_mod2]
  Product4/1 -> [afe_mw_top_mod2]
  Product3/1 -> [afe_mv_bottom_mod2]
  Product2/1 -> [afe_mv_top_mod2]
  Product1/1 -> [afe_mu_bottom_mod2]
  Product/1 -> [afe_mu_top_mod2]
  Bus Selector/6 -> Product5/2  "<gate_cmd_Q6>"
  Bus Selector/5 -> Product4/2  "<gate_cmd_Q5>"
  Bus Selector/4 -> Product3/2  "<gate_cmd_Q4>"
  Bus Selector/3 -> Product2/2  "<gate_cmd_Q3>"
  Bus Selector/2 -> Product1/2  "<gate_cmd_Q2>"
  Bus Selector/1 -> Product/2  "<gate_cmd_Q1>"
  Step/1 -> Product1/1, Product/1, Product2/1, Product3/1, Product4/1, Product5/1
  ileg_dc_inv/1 -> [ileg_dc_afe_mod2]
  ic_dclink/1 -> [ic_dclink_mod2]
  udc/1 -> [udc_mod2]  "udc"
  sv_pwm/1(gate_cmds) -> Bus Selector/1
  [afe_mw_bottom_mod2] -> Simulink-PS Converter5/1
  [afe_mw_top_mod2] -> Simulink-PS Converter4/1
  [afe_mv_bottom_mod2] -> Simulink-PS Converter3/1
  [afe_mv_top_mod2] -> Simulink-PS Converter2/1
  [afe_mu_bottom_mod2] -> Simulink-PS Converter1/1
  [afe_mu_top_mod2] -> Simulink-PS Converter/1
  dabc/1 -> sv_pwm/1(duties_uvw)
  connections:
  Voltage Sensor3/RConn2 -- Electrical Reference2/LConn1
  PS-Simulink Converter2/LConn1 -- Voltage Sensor3/RConn1
  Voltage Sensor1/RConn2 -- Electrical Reference1/LConn1
  PS-Simulink Converter1/LConn1 -- Voltage Sensor1/RConn1
  Voltage Sensor/RConn1 -- PS-Simulink Converter4/LConn1
  Voltage Sensor/RConn2 -- Electrical Reference/LConn1
  Resistor/RConn1 -- Voltage Sensor/LConn1 -- Resistor1/LConn1
  Current Sensor1/RConn1 -- ileg_dc_inv/LConn1
  switch_1/LConn2 -- Current Sensor1/RConn2
  Current Sensor/RConn1 -- ic_dclink/LConn1
  Current Sensor/RConn2 -- Capacitor/LConn1
  dclink_measure/LConn1 -- udc/LConn1 -- Voltage Sensor2/RConn1
  switch_5/RConn1 -- switch_6/LConn2 -- us_c/RConn1
  switch_3/RConn1 -- switch_4/LConn2 -- us_b/RConn1
  switch_1/RConn1 -- switch_2/LConn2 -- us_a/RConn1
  switch_6/LConn1 -- Simulink-PS Converter5/RConn1
  switch_5/LConn1 -- Simulink-PS Converter4/RConn1
  switch_4/LConn1 -- Simulink-PS Converter3/RConn1
  switch_3/LConn1 -- Simulink-PS Converter2/RConn1
  switch_2/LConn1 -- Simulink-PS Converter1/RConn1
  switch_1/LConn1 -- Simulink-PS Converter/RConn1
  switch_4/RConn1 -- switch_6/RConn1 -- switch_2/RConn1 -- Voltage Sensor1/LConn1 -- Resistor1/RConn1 -- Voltage Sensor2/RConn2 -- Capacitor/RConn1 -- Udc(-)/RConn1
  switch_3/LConn2 -- switch_5/LConn2 -- Current Sensor1/LConn1 -- Voltage Sensor3/LConn1 -- Resistor/LConn1 -- Voltage Sensor2/LConn1 -- Udc(+)/RConn1 -- Current Sensor/LConn1

== system afe_abc_inv_psm/afe_abc_inv_psm_mod2/brake ==
  Constant1 : Constant  Value=Vdc_ref
  Current Sensor3 : fl_lib/Electrical/Electrical Sensors/Current Sensor
  Integrator : Integrator
  MATLAB Function : MATLAB Function  TreatAsAtomicUnit=on  SystemSampleTime=ts_afe
  PS-Simulink Converter : nesl_utility/PS-Simulink Converter  PhysicalDomain=network_engine_domain  SubClassName=ps_output  LeftPortType=input  RightPortType=output  PseudoPeriodic=off  Frequencies=[]  VectorFormat=1-D array  Unit=V  AffineConversion=off
  Product : Product
  Product6 : Product
  Rbrake mod2 : Scope  NumInputPorts=2
      settings: SampleTime=tc  ActiveDisplayYMinimum=-1  ActiveDisplayYMaximum=1  DataLoggingVariableName=ScopeData2
  Resistor : fl_lib/Electrical/Electrical Elements/Resistor  R=4 Ohm  i_specify=off  i_priority=None  i=0 A  i_nominal_specify=off  i_nominal_value=1  i_nominal_unit=A  v_specify=off  v_priority=None  v=0 V  v_nominal_specify=off  v_nominal_value=1  v_nominal_unit=V
  Simulink-PS Converter4 : nesl_utility/Simulink-PS Converter  PhysicalDomain=network_engine_domain  SubClassName=ps_input  LeftPortType=input  RightPortType=output  PseudoPeriodic=off  Frequencies=[]  NoiseDistribution=none  NoiseParameters=[]  Unit=1  AffineConversion=on  FilteringAndDerivatives=provide  SimscapeFilterOrder=1  InputFilterTimeConstant=0.001  UdotUserProvided=0
  Step : Step  Time=time_aux_power_supply_fault  Before=1  After=0  SampleTime=0
  To Workspace1 : ToWorkspace  VariableName=energy_Rbrake_sim_mod2  SampleTime=ts_afe
      settings: MaxDataPoints=Ns_afe
  To Workspace10 : ToWorkspace  VariableName=power_Rbrake_sim_mod2  SampleTime=ts_afe
      settings: MaxDataPoints=Ns_afe
  Unit Delay : UnitDelay  SampleTime=ts_afe  HasFrameUpgradeWarning=on
  Voltage Sensor : fl_lib/Electrical/Electrical Sensors/Voltage Sensor
  Voltage Sensor1 : fl_lib/Electrical/Electrical Sensors/Voltage Sensor
  ibrakeR : nesl_utility/PS-Simulink Converter  PhysicalDomain=network_engine_domain  SubClassName=ps_output  LeftPortType=input  RightPortType=output  PseudoPeriodic=off  Frequencies=[]  VectorFormat=1-D array  Unit=A  AffineConversion=off
  switch_5 : Subsystem
      settings: PortSchema="{\"entries\":[{\"content\":{\"sides\":[{\"content\":{\"connectorIds\":[\"LConn1\"]},\"type\":\"ConnectorPlacement.EquallySpacedRectSide\",\"uuid\":\"9277da8d-d460-43e6-8478-dd662f15d226\"},{\"content\":{\"connectorIds\":[],\"side\":\"RIGHT\"},\"type\":\"ConnectorPlacement.EquallySpacedRectSide\",\"uuid\":\"a7ece396-f1d9-4f4f-a05b-db1fc65d6e1d\"},{\"content\":{\"connectorIds\":[\"LConn2\"],\"side\":\"TOP\"},\"type\":\"ConnectorPlacement.EquallySpacedRectSide\",\"uuid\":\"fdd70777-e9cf-4317-afb6-cae87f75d5b0\"},{\"content\":{\"connectorIds\":[\"RConn1\"],\"side\":\"BOTTOM\"},\"type\":\"ConnectorPlacement.EquallySpacedRectSide\",\"uuid\":\"2353ed68-b1a1-4775-9ca9-31e268d5443b\"}]},\"type\":\"ConnectorPlacement.EquallySpacedConnector\",\"uuid\":\"d5479f4c-4e65-4791-adcb-73df11f88590\"}],\"packageUris\":[\"http://schema.mathworks.com/mf0/Connector/R2020b\"],\"version\":\"1.0\"}"
  switch_6 : Subsystem
      settings: PortSchema="{\"entries\":[{\"content\":{\"sides\":[{\"content\":{},\"type\":\"ConnectorPlacement.EquallySpacedRectSide\",\"uuid\":\"9277da8d-d460-43e6-8478-dd662f15d226\"},{\"content\":{\"side\":\"RIGHT\"},\"type\":\"ConnectorPlacement.EquallySpacedRectSide\",\"uuid\":\"a7ece396-f1d9-4f4f-a05b-db1fc65d6e1d\"},{\"content\":{\"connectorIds\":[\"LConn1\"],\"side\":\"TOP\"},\"type\":\"ConnectorPlacement.EquallySpacedRectSide\",\"uuid\":\"fdd70777-e9cf-4317-afb6-cae87f75d5b0\"},{\"content\":{\"connectorIds\":[\"RConn1\"],\"side\":\"BOTTOM\"},\"type\":\"ConnectorPlacement.EquallySpacedRectSide\",\"uuid\":\"2353ed68-b1a1-4775-9ca9-31e268d5443b\"}]},\"type\":\"ConnectorPlacement.EquallySpacedConnector\",\"uuid\":\"d5479f4c-4e65-4791-adcb-73df11f88590\"}],\"packageUris\":[\"http://schema.mathworks.com/mf0/Connector/R2020b\"],\"version\":\"1.0\"}"
  ubrakeR : nesl_utility/PS-Simulink Converter  PhysicalDomain=network_engine_domain  SubClassName=ps_output  LeftPortType=input  RightPortType=output  PseudoPeriodic=off  Frequencies=[]  VectorFormat=1-D array  Unit=V  AffineConversion=off
  dc(+) : PMIOPort  Side=Left
  dc(-) : PMIOPort  Port=2  Side=Left
  tag scope: energy_Rbrake_mod2=global, power_Rbrake_mod2=global
  wires:
  Product6/1 -> Simulink-PS Converter4/1
  Unit Delay/1 -> Product6/2
  Step/1 -> Product6/1
  [energy_Rbrake_mod2] -> Rbrake mod2/2, To Workspace1/1  "energy_Rbrake"
  [power_Rbrake_mod2] -> Rbrake mod2/1, To Workspace10/1  "power_Rbrake"
  Integrator/1 -> [energy_Rbrake_mod2]
  Product/1 -> Integrator/1, [power_Rbrake_mod2]
  ubrakeR/1 -> Product/2  "ubrakeR"
  ibrakeR/1 -> Product/1  "ibrakeR"
  MATLAB Function/1(y) -> Unit Delay/1
  PS-Simulink Converter/1 -> MATLAB Function/1(u)
  Constant1/1 -> MATLAB Function/2(udc_ref)
  connections:
  Voltage Sensor1/RConn1 -- ubrakeR/LConn1
  Current Sensor3/RConn1 -- ibrakeR/LConn1
  dc(+)/RConn1 -- switch_6/LConn1 -- Current Sensor3/LConn1 -- Voltage Sensor/LConn1
  switch_5/LConn2 -- Resistor/RConn1 -- Voltage Sensor1/RConn2 -- switch_6/RConn1
  switch_5/LConn1 -- Simulink-PS Converter4/RConn1
  PS-Simulink Converter/LConn1 -- Voltage Sensor/RConn1
  Current Sensor3/RConn2 -- Resistor/LConn1 -- Voltage Sensor1/LConn1
  Voltage Sensor/RConn2 -- switch_5/RConn1 -- dc(-)/RConn1

== system afe_abc_inv_psm/afe_abc_inv_psm_mod2/inverter ==
  duvw : Inport
  Current Sensor : fl_lib/Electrical/Electrical Sensors/Current Sensor
  PS-Simulink Converter1 : nesl_utility/PS-Simulink Converter  PhysicalDomain=network_engine_domain  SubClassName=ps_output  LeftPortType=input  RightPortType=output  PseudoPeriodic=off  Frequencies=[]  VectorFormat=1-D array  Unit=A  AffineConversion=on
  PS-Simulink Converter4 : nesl_utility/PS-Simulink Converter  PhysicalDomain=network_engine_domain  SubClassName=ps_output  LeftPortType=input  RightPortType=output  PseudoPeriodic=off  Frequencies=[]  VectorFormat=1-D array  Unit=V  AffineConversion=on
  To Workspace : ToWorkspace  VariableName=idc_sim_mod2  SampleTime=tc
      settings: MaxDataPoints=Nc
  To Workspace1 : ToWorkspace  VariableName=udc_sim_mod2  SampleTime=tc
      settings: MaxDataPoints=Nc
  Transfer Fcn : TransferFcn  Denominator=[1e-2 1]
  Voltage Sensor : fl_lib/Electrical/Electrical Sensors/Voltage Sensor
  idc/udc mod2 : Scope  NumInputPorts=2
      settings: SampleTime=tc  ActiveDisplayYMinimum=-232.79227304961765  ActiveDisplayYMaximum=27.545875945686063
  inverter : Subsystem
  Udc(+) : PMIOPort  Side=Right
  Udc(-) : PMIOPort  Port=2  Side=Right
  us_u : PMIOPort  Port=3  Side=Left
  us_v : PMIOPort  Port=4  Side=Left
  us_w : PMIOPort  Port=5  Side=Left
  wires:
  duvw/1 -> inverter/1(duties_uvw)
  Transfer Fcn/1 -> idc/udc mod2/1, To Workspace/1  "idc_flt"
  PS-Simulink Converter1/1 -> Transfer Fcn/1  "idc"
  PS-Simulink Converter4/1 -> idc/udc mod2/2, To Workspace1/1  "udc"
  connections:
  PS-Simulink Converter1/LConn1 -- Current Sensor/RConn1
  Current Sensor/RConn2 -- inverter/RConn1 -- Voltage Sensor/LConn1
  Current Sensor/LConn1 -- Udc(+)/RConn1
  Udc(-)/RConn1 -- inverter/RConn2 -- Voltage Sensor/RConn2
  us_w/RConn1 -- inverter/LConn3
  us_v/RConn1 -- inverter/LConn2
  us_u/RConn1 -- inverter/LConn1
  PS-Simulink Converter4/LConn1 -- Voltage Sensor/RConn1

== system afe_abc_inv_psm/global timing/time_afe1 ==
  correction_time : Inport
  Constant : Constant
  Gain : Gain  Gain=k
  Product : Product
  Sum : Sum  Inputs=|++
  time_1 : Clock
  Out1 : Outport
  wires:
  time_1/1 -> Gain/1
  Gain/1 -> Product/1
  Product/1 -> Out1/1
  correction_time/1 -> Sum/1
  Sum/1 -> Product/2
  Constant/1 -> Sum/2

== system afe_abc_inv_psm/global timing/time_afe2 ==
  correction_time : Inport
  Constant : Constant
  Gain : Gain  Gain=k
  Product : Product
  Sum : Sum  Inputs=|++
  time_1 : Clock
  Out1 : Outport
  wires:
  time_1/1 -> Gain/1
  Gain/1 -> Product/1
  Product/1 -> Out1/1
  correction_time/1 -> Sum/1
  Constant/1 -> Sum/2
  Sum/1 -> Product/2

== system afe_abc_inv_psm/global timing/time_afe3 ==
  Gain : Gain  Gain=k
  time_1 : Clock
  Out1 : Outport
  wires:
  Gain/1 -> Out1/1
  time_1/1 -> Gain/1

== system afe_abc_inv_psm/global timing/time_inv1 ==
  correction_time : Inport
  Constant : Constant
  Gain : Gain  Gain=k
  Product : Product
  Sum : Sum  Inputs=|++
  time_1 : Clock
  Out1 : Outport
  wires:
  time_1/1 -> Gain/1
  Gain/1 -> Product/1
  Product/1 -> Out1/1
  correction_time/1 -> Sum/1
  Constant/1 -> Sum/2
  Sum/1 -> Product/2

== system afe_abc_inv_psm/global timing/time_inv2 ==
  correction_time : Inport
  Constant : Constant
  Gain : Gain  Gain=k
  Product : Product
  Sum : Sum  Inputs=|++
  time_1 : Clock
  Out1 : Outport
  wires:
  time_1/1 -> Gain/1
  Gain/1 -> Product/1
  Product/1 -> Out1/1
  correction_time/1 -> Sum/1
  Constant/1 -> Sum/2
  Sum/1 -> Product/2

== system afe_abc_inv_psm/grid/grid_emulator ==
  3ph_Dyg : Subsystem
  Controlled Voltage Source : fl_lib/Electrical/Electrical Sources/Controlled Voltage Source
  Controlled Voltage Source1 : fl_lib/Electrical/Electrical Sources/Controlled Voltage Source
  Controlled Voltage Source2 : fl_lib/Electrical/Electrical Sources/Controlled Voltage Source
  Electrical Reference : fl_lib/Electrical/Electrical Elements/Electrical Reference
  Simulink-PS Converter : nesl_utility/Simulink-PS Converter  PhysicalDomain=network_engine_domain  SubClassName=ps_input  LeftPortType=input  RightPortType=output  PseudoPeriodic=off  Frequencies=[]  NoiseDistribution=none  NoiseParameters=[]  Unit=V  AffineConversion=on  FilteringAndDerivatives=provide  SimscapeFilterOrder=1  InputFilterTimeConstant=0.001  UdotUserProvided=0
  Simulink-PS Converter1 : nesl_utility/Simulink-PS Converter  PhysicalDomain=network_engine_domain  SubClassName=ps_input  LeftPortType=input  RightPortType=output  PseudoPeriodic=off  Frequencies=[]  NoiseDistribution=none  NoiseParameters=[]  Unit=V  AffineConversion=on  FilteringAndDerivatives=provide  SimscapeFilterOrder=1  InputFilterTimeConstant=0.001  UdotUserProvided=0
  Simulink-PS Converter2 : nesl_utility/Simulink-PS Converter  PhysicalDomain=network_engine_domain  SubClassName=ps_input  LeftPortType=input  RightPortType=output  PseudoPeriodic=off  Frequencies=[]  NoiseDistribution=none  NoiseParameters=[]  Unit=V  AffineConversion=on  FilteringAndDerivatives=provide  SimscapeFilterOrder=1  InputFilterTimeConstant=0.001  UdotUserProvided=0
  Solver Configuration : nesl_utility/Solver Configuration  PhysicalDomain=network_engine_domain  SubClassName=solver  LeftPortType=input  RightPortType=generic  Tones=[]  Harmonics=[]  SimulateNoise=off  Profile=off  UseLocalSampling=off  EnableSwitchedLinearOptims=on  FrequencyDomain=off  UseCCode=off  RelTol=0.001  AbsTol=0.001  MinStep=1e-09  ToWorkspace=off  RevertToSquareIcSolve=off  NumHomotopyIterations=100  PhasorMode=off  PhasorModeNumHarmonics=1  ConsistencySolver=NEWTON_FTOL  IndexReductionMethod=DerivativeReplacement  DoDC=off  ResidualTolerance=1e-09  ConsistencyTolSource=GLOBAL  ConsistencyAbsTol=0.001  ConsistencyRelTol=0.001  ConsistencyTolFactor=0.001  UseLocalSolver=on  LocalSolverChoice=NE_BACKWARD_EULER_ADVANCER  ResolveIndetEquations=on  FunctionEvalNumThread=1  LocalSolverSampleTime=tc  DoFixedCost=on  MaxNonlinIter=3  MaxModeIter=2  ComputeImpulses=off  ImpulseIterations=2  LinearAlgebra=auto  LinearAlgebraNumThread=0  EquationFormulation=NE_TIME_EF  DelaysMemoryBudget=1024  AutomaticFiltering=on  FilteringTimeConstant=0.001  PartitionStorageMethod=AS_NEEDED  PartitionMemoryBudget=1024  PartitionMethod=ROBUST  MultibodyUseLocalSolver=off  MultibodyLocalSolverChoice=ODE1  MultibodyLocalSolverSampleTime=0.001
  grid_emulator : Subsystem
  threephase_vi_measures : Subsystem
  u1 : PMIOPort  Side=Right
  u2 : PMIOPort  Port=2  Side=Right
  u3 : PMIOPort  Port=3  Side=Right
  wires:
  grid_emulator/2(Vmb) -> Simulink-PS Converter1/1
  grid_emulator/3(Vmc) -> Simulink-PS Converter2/1
  grid_emulator/1(Vma) -> Simulink-PS Converter/1
  connections:
  Simulink-PS Converter/RConn1 -- Controlled Voltage Source/RConn1
  Simulink-PS Converter1/RConn1 -- Controlled Voltage Source1/RConn1
  Simulink-PS Converter2/RConn1 -- Controlled Voltage Source2/RConn1
  Electrical Reference/LConn1 -- Solver Configuration/RConn1 -- Controlled Voltage Source/RConn2 -- Controlled Voltage Source1/RConn2 -- Controlled Voltage Source2/RConn2
  3ph_Dyg/RConn1 -- u1/RConn1
  3ph_Dyg/RConn2 -- u2/RConn1
  3ph_Dyg/RConn3 -- u3/RConn1
  threephase_vi_measures/RConn1 -- 3ph_Dyg/LConn1
  threephase_vi_measures/RConn2 -- 3ph_Dyg/LConn2
  threephase_vi_measures/RConn3 -- 3ph_Dyg/LConn3
  Controlled Voltage Source/LConn1 -- threephase_vi_measures/LConn1
  Controlled Voltage Source1/LConn1 -- threephase_vi_measures/LConn2
  Controlled Voltage Source2/LConn1 -- threephase_vi_measures/LConn3
